simulink model "RNN_MAC"  (R2020b)
settings: Solver=VariableStepAuto  StartTime=0.0  StopTime=10.0  RelTol=1e-3
undefined symbols (not defined in the file): a, b, c
libraries: hdlsllib x2
settings Model: Creator=chank  LastModifiedBy=chank

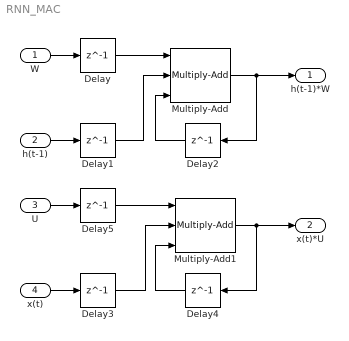
== system RNN_MAC ==
  W : Inport  OutDataTypeStr=single
  h(t-1) : Inport  Port=2  OutDataTypeStr=single
  U : Inport  Port=3  OutDataTypeStr=single
  x(t) : Inport  Port=4  OutDataTypeStr=single
  Delay{,1..5} (6 alike) : Delay  DelayLength=1
  Multiply-Add : hdlsllib/HDL Operations/Multiply-Add  Function=c+(a.*b)  datatype=Inherit: Inherit via internal rule  DoSatur=off  FMA=off
      settings: SourceProductBaseCode=SL
  Multiply-Add1 : hdlsllib/HDL Operations/Multiply-Add  Function=c+(a.*b)  datatype=Inherit: Inherit via internal rule  DoSatur=off  FMA=off
      settings: SourceProductBaseCode=SL
  h(t-1)*W : Outport
  x(t)*U : Outport  Port=2
  wires:
  W/1 -> Delay/1
  h(t-1)/1 -> Delay1/1
  x(t)/1 -> Delay3/1
  U/1 -> Delay5/1
  Delay/1 -> Multiply-Add/1
  Delay1/1 -> Multiply-Add/2
  Delay2/1 -> Multiply-Add/3
  Multiply-Add/1 -> Delay2/1, h(t-1)*W/1
  Delay5/1 -> Multiply-Add1/1
  Delay3/1 -> Multiply-Add1/2
  Delay4/1 -> Multiply-Add1/3
  Multiply-Add1/1 -> Delay4/1, x(t)*U/1
